simulink model "es1_01"  (R2020a)
settings: Solver=VariableStepAuto  StartTime=0.0  StopTime=10.0  MaxStep=0.01  RelTol=1e-3
undefined symbols (not defined in the file): A, B, C, D
settings Model: Creator=EREN  LastModifiedBy=EREN

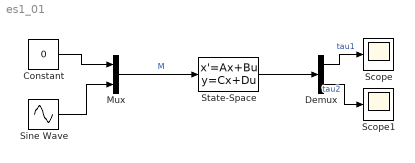
== system es1_01 ==
  Constant : Constant  Value=0
  Demux : Demux  Outputs=2
  Mux : Mux  Inputs=2
  Scope : Scope
  Scope1 : Scope
  Sine Wave : Sin  Amplitude=100  Frequency=8  SampleTime=0
  State-Space : StateSpace  A=A  B=B  C=C  D=D  InitialCondition=0
  wires:
  State-Space/1 -> Demux/1
  Demux/1 -> Scope/1  "tau1"
  Demux/2 -> Scope1/1  "tau2"
  Mux/1 -> State-Space/1  "M"
  Sine Wave/1 -> Mux/2
  Constant/1 -> Mux/1
